simulink library "lib_torque_limit_calculator"  (R2023a)
settings: Solver=VariableStepAuto  StartTime=0.0  StopTime=10.0  RelTol=1e-3
undefined symbols (not defined in the file): bit
libraries: lib_discrete_time_integrator x1, simulink x1
settings Model: Creator=cav2ofo  LastModifiedBy=lenovo
settings OptimizationCC: ReuseModelBlockBuffer=off

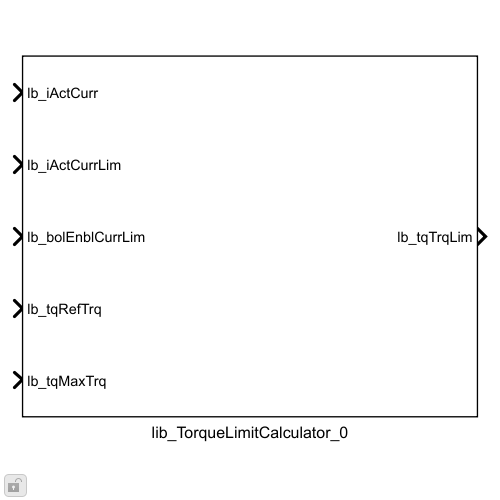
[thumbnail: Simulink's stored preview of the top-level diagram]
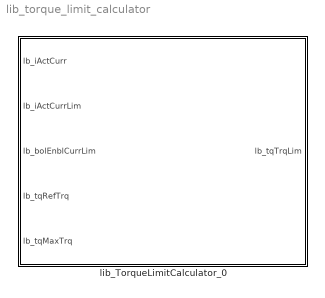
== system lib_torque_limit_calculator ==
  lib_TorqueLimitCalculator_0 : Subsystem  mask{lb_parSampTime=0.01, lb_parMaxSampTime=0.01, lb_parIntgGain=0, lb_parMaxIntgGain=1, lb_parMaxInpVal=50, lb_parMinInpVal=-1, lb_parIntgScopMode=Integral control, lb_parSatFlag=on, lb_parAccmDataTypeMode=32-bit, lb_parOutpDataType=fixdt(1,16,2^-14,0)}
      mask prompts: lb_parSampTime "Sampling time [s]:"; lb_parMaxSampTime "Maximum sampling time [s]:"; lb_parIntgGain "Integral gain [Nm*s/A]:"; lb_parMaxIntgGain "Maximum integral gain [Nm*s/A]:"; lb_parMaxInpVal "Maximum current margin [A]:"; lb_parMinInpVal "Minimum current margin [A]:"; lb_parIntgScopMode "Integration scope:"; lb_parSatFlag "Output saturation"; lb_parAccmDataTypeMode "Accumulator data type mode:"; lb_parOutpDataType "Output data type:"
      mask init:
      | lb_parMaxSampTime = double(lb_parSampTime);
      | lb_parMinInpVal = -double(lb_parMaxInpVal);
      mask TypeOptions lb_parMaxSampTime: lib_DiscreteTimeIntegrator_1/lb_parMaxSampTime
      mask TypeOptions lb_parMaxIntgGain: lib_DiscreteTimeIntegrator_1/lb_parMaxIntgGain
      mask TypeOptions lb_parMaxInpVal: lib_DiscreteTimeIntegrator_1/lb_parMaxInpVal
      mask TypeOptions lb_parMinInpVal: lib_DiscreteTimeIntegrator_1/lb_parMinInpVal
      mask TypeOptions lb_parIntgScopMode: lib_DiscreteTimeIntegrator_1/lb_parIntgScopMode
      mask TypeOptions lb_parSatFlag: lib_DiscreteTimeIntegrator_1/lb_parSatFlag
      mask TypeOptions lb_parAccmDataTypeMode: lib_DiscreteTimeIntegrator_1/lb_parAccmDataTypeMode
      mask TypeOptions lb_parOutpDataType: lib_DiscreteTimeIntegrator_1/lb_parOutpDataType
      mask DialogControl Container2 Prompt: VHIT control library
      mask DialogControl Control1 Prompt: Torque limit calculator
      mask DialogControl Container1 Prompt: Parameters
      mask DialogControl Container3 Prompt: Operating modes:
      mask DialogControl Container4 Prompt: Data types

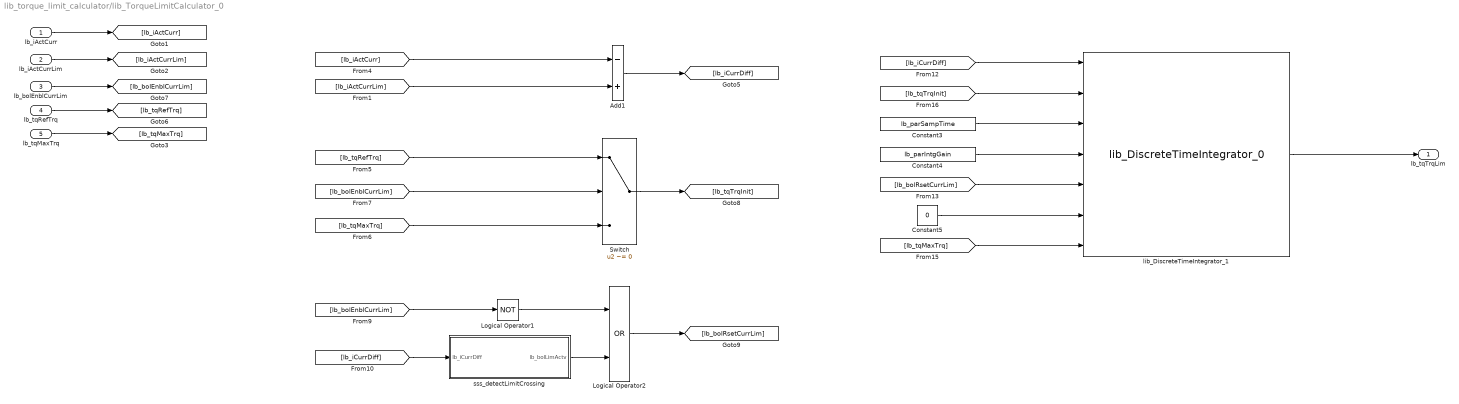
== system lib_torque_limit_calculator/lib_TorqueLimitCalculator_0 ==
  lb_iActCurr : Inport
  lb_iActCurrLim : Inport  Port=2
  lb_bolEnblCurrLim : Inport  Port=3
  lb_tqRefTrq : Inport  Port=4
  lb_tqMaxTrq : Inport  Port=5
  Add1 : Sum  Inputs=-+  RndMeth=Simplest  OutDataTypeStr=Inherit: Same as first input
  Constant3 : Constant  Value=lb_parSampTime
  Constant4 : Constant  Value=lb_parIntgGain
  Constant5 : Constant  Value=0  OutDataTypeStr=lb_parOutpDataType
  Logical Operator1 : Logic  Operator=NOT  AllPortsSameDT=off  OutDataTypeStr=boolean
  Logical Operator2 : Logic  Operator=OR  AllPortsSameDT=off  OutDataTypeStr=boolean
  Switch : Switch  Criteria=u2 ~= 0  SaturateOnIntegerOverflow=off  InputSameDT=off
  lib_DiscreteTimeIntegrator_1 : lib_discrete_time_integrator/lib_DiscreteTimeIntegrator_0  lb_parMaxInpVal=lb_parMaxInpVal  lb_parMinInpVal=lb_parMinInpVal  lb_parMaxSampTime=lb_parMaxSampTime  lb_parMaxIntgGain=lb_parMaxIntgGain  lb_parAccmDataTypeMode=32-bit  lb_parOutpDataType=fixdt(1,16,2^-14,0)  lb_parIntgScopMode=Integral control  lb_parSatFlag=on
      settings: LibrarySourceBlock=vhit_control_library/lib_DiscreteTimeIntegrator_0
  sss_detectLimitCrossing : Subsystem
  lb_tqTrqLim : Outport
  wires:
  lib_DiscreteTimeIntegrator_1/1 -> lb_tqTrqLim/1
  lb_iActCurr/1 -> [lb_iActCurr]
  lb_iActCurrLim/1 -> [lb_iActCurrLim]
  lb_tqMaxTrq/1 -> [lb_tqMaxTrq]
  [lb_iActCurr] -> Add1/1
  [lb_iActCurrLim] -> Add1/2
  Add1/1 -> [lb_iCurrDiff]
  lb_tqRefTrq/1 -> [lb_tqRefTrq]
  lb_bolEnblCurrLim/1 -> [lb_bolEnblCurrLim]
  [lb_bolEnblCurrLim] -> Switch/2
  Switch/1 -> [lb_tqTrqInit]
  [lb_bolEnblCurrLim] -> Logical Operator1/1
  Logical Operator1/1 -> Logical Operator2/1
  Logical Operator2/1 -> [lb_bolRsetCurrLim]
  [lb_tqRefTrq] -> Switch/1
  [lb_tqMaxTrq] -> Switch/3
  [lb_iCurrDiff] -> sss_detectLimitCrossing/1(lb_iCurrDiff)
  sss_detectLimitCrossing/1(lb_bolLimActv) -> Logical Operator2/2
  [lb_iCurrDiff] -> lib_DiscreteTimeIntegrator_1/1
  Constant5/1 -> lib_DiscreteTimeIntegrator_1/6
  [lb_bolRsetCurrLim] -> lib_DiscreteTimeIntegrator_1/5
  Constant3/1 -> lib_DiscreteTimeIntegrator_1/3
  [lb_tqTrqInit] -> lib_DiscreteTimeIntegrator_1/2
  [lb_tqMaxTrq] -> lib_DiscreteTimeIntegrator_1/7
  Constant4/1 -> lib_DiscreteTimeIntegrator_1/4

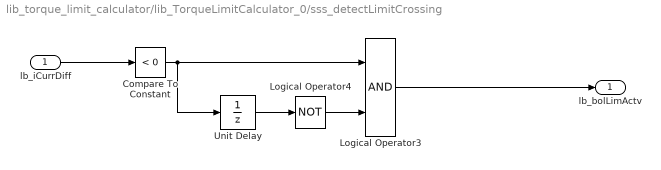
== system lib_torque_limit_calculator/lib_TorqueLimitCalculator_0/sss_detectLimitCrossing ==
  lb_iCurrDiff : Inport
  Compare To Constant : simulink/Logic and Bit Operations/Compare To Constant  relop=<  const=0  OutDataTypeStr=boolean
  Logical Operator3 : Logic  AllPortsSameDT=off  OutDataTypeStr=boolean
  Logical Operator4 : Logic  Operator=NOT  AllPortsSameDT=off  OutDataTypeStr=boolean
  Unit Delay : UnitDelay  SampleTime=-1  HasFrameUpgradeWarning=on
  lb_bolLimActv : Outport
  wires:
  Logical Operator3/1 -> lb_bolLimActv/1
  lb_iCurrDiff/1 -> Compare To Constant/1
  Logical Operator4/1 -> Logical Operator3/2
  Unit Delay/1 -> Logical Operator4/1
  Compare To Constant/1 -> Unit Delay/1, Logical Operator3/1
